simulink model "V1"  (R2025a)
settings: Solver=VariableStepAuto  StartTime=0.0  StopTime=200  FixedStep=0.005  RelTol=1e-3
libraries: cstblocks x11, vrlib x10, slpidlib x9, simulink_extras x8, dspinverses x3, robotcorelib x2, simulink x1
(part 1 of 3)
settings Model: Creator=HyeonMin  LastModifiedBy=user
settings SolverCC: AlgebraicLoopSolver=TrustRegion
settings DebuggingCC: UnderSpecifiedDimensionMsg=warning
settings RTWCC: GPUComputeCapability=3.5

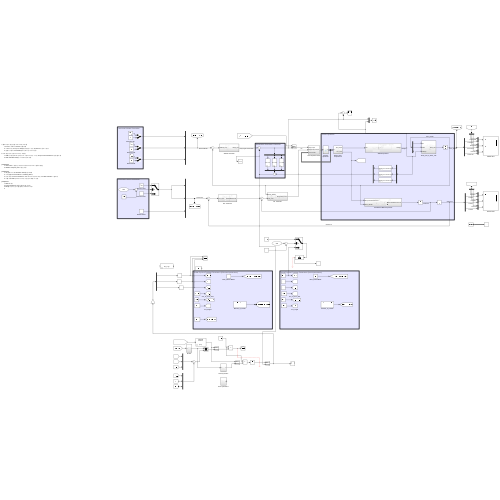
[thumbnail: Simulink's stored preview of the top-level diagram]
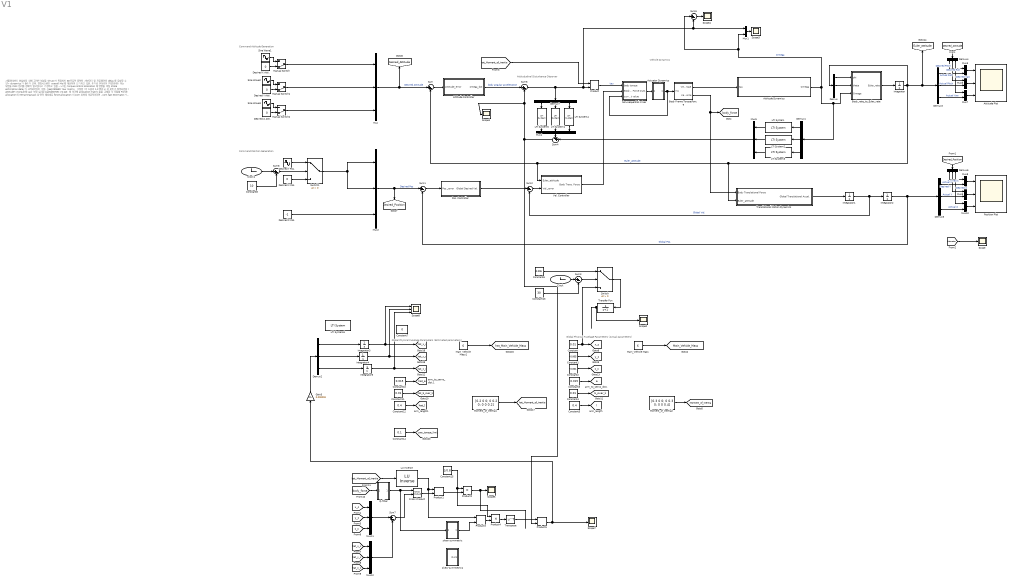
== system V1 ==
  note: Attitududinal Disturbance Observer
  note: Command Attitude Generation
  note: Command Position Generation
  note: 시뮬레이션의 현실성을 위해 고려한 부분들
      | thrust가 목표치의 80프로만 출력됨
      | 서보모터 및 프로펠러에 delay를 유발할 수 있는 dynamics가 들어가 있음.
      | 결합시스템의 overall MoI를 계산하여 인가하고 있음.
      |
      | 추가로 현실성이 반영되어야 하는 부분들
      | CoM 텐서를 정확히 알고있다고 가정하고 있음. ->이는 torque control allocation에 영향을 미침
      | state estimation delay가 고려되어있지 않음.
      |
      | [Jae]230630:
      | Yaw matrix 수정함 (각 드론의 1,2행의 xi 값 부호가 잘못되었음)
      | attitude->torque에 yaw 보정 실시함
      |
      | [Jae]230705:
      | V2 ppt에 의거해 allocation matrix들을 교체함
      | 각 모듈별 Force allocation이 remaining task임
      | 만약 예상대로 force allocation이 com 위치에 의존적이라면, com fast estimator가 필요함
      | 이를 위해 DOB 신호에 의거하는 것을 생각해볼 수 있음.
      |
      | [Jae]230731:
      | DOB 추가함.
      | torque allocation을 J를 곱함으로써 추가함.
      | MoI를 계산하는 공식을 물리량 파트에 추가함.
  note: Global Physical Fuselage Parameters (Actual parameters)
  note: Vehicle Dynamics
  note: Global Physical Fuselage Parameters (Estimated parameters)
  " LU Inverse" : dspinverses/ LU Inverse
  Actuator Dynamics : Subsystem
  Attitude Controller : Subsystem
  Attitude Dynamics : Subsystem
  Attitude Plot : Scope  NumInputPorts=3
      settings: Title=Fuselage Euler Attitude  ActiveDisplayYMinimum=-0.24923  ActiveDisplayYMaximum=0.11713  YLabel=Roll
  Body Frame Torque/Force : Subsystem
  Body_rate_to_Euler_rate : Subsystem
  Clock : Clock
  Clock1 : Clock
  Constant : Constant  Value=0.01
  Constant1 : Constant  Value=-0.005
  Constant10 : Constant  Value=0.015
  Constant11 : Constant  Value=0.01
  Constant12 : Constant  Value=0.4
  Constant13 : Constant  Value=30
  Constant14 : Constant  Value=0.1
  Constant15 : Constant  Value=1/0.8
  Constant2 : Constant  Value=-0.001
  Constant3 : Constant  Value=0.015
  Constant4 : Constant  Value=0.01
  Constant5 : Constant  Value=0.4
  Constant6 : Constant  Value=0.005
  Constant7 : Constant  Value=0
  Constant8 : Constant  Value=10
  Cross Product : vrlib/Utilities/Cross Product
  Demux{,1..7} (8 alike) : Demux  Outputs=3
  Desired X Atti. : Constant  Value=0
  Desired X Pos. : Constant  Value=0
  Desired Y Atti. : Constant  Value=0
  Desired Y Pos. : Sin  Amplitude=10  Frequency=0.5  SampleTime=0
  Desired Z Atti. : Constant  Value=0
  Desired Z Pos. : Constant  Value=-1
  Gain3 : Gain  Gain=0.000003
  Integrator{,1..5} (6 alike) : Integrator
  LTI System : cstblocks/LTI System  sys=tf([1 0],[1/1 1.414/1 1])  IC=[]  PadeOrder=0
  LTI System1 : cstblocks/LTI System  sys=tf([1],[1/1 1.414/1 1])  IC=[]  PadeOrder=0
  LTI System2 : cstblocks/LTI System  sys=tf([1 0],[1/1 1.414/1 1])  IC=[]  PadeOrder=0
  LTI System3 : cstblocks/LTI System  sys=tf([1 0],[1/1 1.414/1 1])  IC=[]  PadeOrder=0
  LTI System4 : cstblocks/LTI System  sys=tf([1],[1/1 1.414/1 1])  IC=[]  PadeOrder=0
  LTI System5 : cstblocks/LTI System  sys=tf([1],[1/1 1.414/1 1])  IC=[]  PadeOrder=0
  LTI System6 : cstblocks/LTI System  sys=tf(1,[1 1])  IC=[]  PadeOrder=0
  Main_Vehicle Mass : Constant  Value=6
  Main_Vehicle Mass1 : Constant  Value=6
  Manual Switch : ManualSwitch  CurrentSetting=0
  Manual Switch1 : ManualSwitch  CurrentSetting=0
  Manual Switch2 : ManualSwitch  CurrentSetting=0
  Moment_of_Inertia1 : Constant  Value=[0.2 0 0; 0 0.2 0; 0 0 0.2]  VectorParams1D=off
  Moment_of_Inertia2 : Constant  Value=[0.3 0 0; 0 0.3 0; 0 0 0.4]  VectorParams1D=off
  Mux{,2,4..5,11..12} (6 alike) : Mux  Inputs=3
  Mux{1,3,6..10} (7 alike) : Mux  Inputs=2
  Non-sequential mixer : Subsystem
  Pos. Controller : Subsystem
  Position Plot : Scope  NumInputPorts=3
      settings: Title=Fuselage Global Position  ActiveDisplayYMinimum=-12.5  ActiveDisplayYMaximum=12.5  YLabel=X Pos.
  Product{,1,3,5} (4 alike) : Product  Multiplication=Matrix(*)
  Product2 : Product
  Product4 : Product
  Q-filter : Subsystem
  Scope{,1..5,7} (7 alike) : Scope
      Scope settings: ActiveDisplayYMinimum=-12.2499  ActiveDisplayYMaximum=102.16663  DataLoggingVariableName=ScopeData2
      Scope1 settings: ActiveDisplayYMinimum=-1.84038  ActiveDisplayYMaximum=0.46914
      Scope2 settings: ActiveDisplayYMinimum=-0.00062  ActiveDisplayYMaximum=0.00562  DataLoggingVariableName=ScopeData7
      Scope3 settings: ActiveDisplayYMinimum=-16.98597  ActiveDisplayYMaximum=13.16908  DataLoggingVariableName=ScopeData2
      Scope4 settings: ActiveDisplayYMinimum=-12.97439  ActiveDisplayYMaximum=18.15104  DataLoggingVariableName=ScopeData3
      Scope5 settings: ActiveDisplayYMinimum=-11.747663892139656  ActiveDisplayYMaximum=3.3030131405781913  DataLoggingVariableName=ScopeData4
      Scope7 settings: ActiveDisplayYMinimum=-1130.28192  ActiveDisplayYMaximum=1419.66244  DataLoggingVariableName=ScopeData6
  Scope8 : Scope  NumInputPorts=3
      settings: ActiveDisplayYMinimum=-0.00763  ActiveDisplayYMaximum=0.01321  DataLoggingVariableName=ScopeData7
  Sine Wave1 : Sin  Amplitude=0.2  Frequency=0.4  SampleTime=0
  Sine Wave2 : Sin  Amplitude=0.2  Frequency=0.4  SampleTime=0
  Sine Wave3 : Sin  Frequency=0.2  SampleTime=0
  Sum{,1..3,5..8} (8 alike) : Sum  Inputs=|+-
  Sum4 : Sum  Inputs=-+|
  Switch : Switch  Criteria=u2 > Threshold  SaturateOnIntegerOverflow=off  InputSameDT=off
  Switch1 : Switch  Criteria=u2 > Threshold  SaturateOnIntegerOverflow=off  InputSameDT=off
  Transfer Fcn : TransferFcn  Denominator=[1 1]
  Translational Motion Dynamics : Subsystem
  Transpose : Math  Operator=transpose
  Vel. Controller : Subsystem
  skew-symmetric : Subsystem
  skew-symmetric1 : Subsystem
  tag scope: Desired_Attitude=global, Desired_Position=global, Euler_attitude=global, Main_Vehicle_Mass=global, Moment_of_Inertia=global, a=global, b_over_k=global, body_force=global, hat_Main_Vehicle_Mass=global, hat_Moment_of_Inertia=global, hat_a=global, hat_b_over_k=global, hat_l=global, hat_x_c=global, hat_y_c=global, hat_z_c=global, l=global, x_c=global, y_c=global, yaw_torque_limit=global, z_c=global
  wires:
  Mux/1 -> Sum/1, [Desired_Attitude]  "Desired Attitude"
  Sum/1 -> Attitude Controller/1(Attitude_error)
  Mux2/1 -> Sum1/1, [Desired_Position]  "Desired Pos"
  Desired Z Pos./1 -> Mux2/3
  Sum1/1 -> Pos. Controller/1(Pos._error)
  Pos. Controller/1(Global Desired Vel.) -> Sum2/1
  Sum2/1 -> Vel. Controller/2(Vel._error)
  Constant/1 -> [x_c], Switch/3
  Constant1/1 -> [y_c]
  Constant2/1 -> [z_c]
  Constant3/1 -> [a]
  Constant4/1 -> [b_over_k]
  Constant5/1 -> [l]
  Main_Vehicle Mass/1 -> [Main_Vehicle_Mass]
  Non-sequential mixer/1(Out1) -> Actuator Dynamics/1(In1)
  Integrator/1 -> Translational Motion Dynamics/2(Euler_attitude), Sum/2, Vel. Controller/1(Euler_attitude), [Euler_attitude], Demux3/1, Demux/1  "Euler_attitude"
  Demux/2 -> Body_rate_to_Euler_rate/2(theta)
  Demux/1 -> Body_rate_to_Euler_rate/1(phi)
  Demux4/1 -> Mux3/1  "Desired Roll"
  Demux4/2 -> Mux6/1  "Desired Pitch"
  [Desired_Attitude] -> Demux4/1
  Demux3/3 -> Mux7/2  "Actual Yaw"
  Demux3/1 -> Mux3/2  "Actual Roll"
  Demux3/2 -> Mux6/2  "Actual Pitch"
  Demux4/3 -> Mux7/1  "Desired Yaw"
  Mux3/1 -> Attitude Plot/1
  Mux6/1 -> Attitude Plot/2
  Mux7/1 -> Attitude Plot/3
  Body Frame Torque/Force/2(Vec_force) -> [body_force], Translational Motion Dynamics/1(Body Translational Force)
  Demux6/1 -> Mux8/1  "Desired X"
  Demux5/3 -> Mux10/2  "Actual Z"
  [Desired_Position] -> Demux6/1
  Mux9/1 -> Position Plot/2
  Demux6/3 -> Mux10/1  "Desired Z"
  Demux6/2 -> Mux9/1  "Desired Y"
  Demux5/1 -> Mux8/2  "Actual X"
  [Actuator] -> Scope/1
  Demux5/2 -> Mux9/2  "Actual Y"
  Mux8/1 -> Position Plot/1
  Integrator2/1 -> Sum1/2, Demux5/1  "Global Pos."
  Mux10/1 -> Position Plot/3
  Translational Motion Dynamics/1(Global Translational Accel.) -> Integrator1/1
  Integrator1/1 -> Sum2/2, Integrator2/1  "Global Vel."
  Sine Wave1/1 -> Manual Switch/1
  Manual Switch/1 -> Mux/1
  Sine Wave3/1 -> Manual Switch2/1
  Manual Switch2/1 -> Mux/3
  Desired X Atti./1 -> Manual Switch/2
  Sine Wave2/1 -> Manual Switch1/1
  Desired Y Atti./1 -> Manual Switch1/2
  Desired Z Atti./1 -> Manual Switch2/2
  Manual Switch1/1 -> Mux/2
  Attitude Dynamics/1(Omega) -> Sum5/1, Mux1/2, Demux1/1, Body_rate_to_Euler_rate/3(Omega)  "Omega"
  Actuator Dynamics/1(Out1) -> Non-sequential mixer/3(current value), Body Frame Torque/Force/1(In1)
  Main_Vehicle Mass1/1 -> [hat_Main_Vehicle_Mass]
  Constant12/1 -> [hat_l]
  Demux2/3 -> Integrator5/1
  Demux2/1 -> Integrator3/1
  Demux2/2 -> Integrator4/1
  Constant11/1 -> [hat_b_over_k]
  Constant10/1 -> [hat_a]
  Body Frame Torque/Force/1(Vec_torque) -> Attitude Dynamics/1(tau)
  Sum6/1 -> Sum5/2, Mux1/1, Product/2, Demux7/1
  Vel. Controller/1(Body Trans. Force) -> Non-sequential mixer/2(Body Trans. Force)
  Constant14/1 -> [yaw_torque_limit]
  [hat_Moment_of_Inertia] -> Product/1
  Product/1 -> Non-sequential mixer/1(body torque)  "tau"
  Attitude Controller/1(omega_dot) -> Sum6/1  "body angular acceleration"
  Moment_of_Inertia1/1 -> [hat_Moment_of_Inertia]
  Moment_of_Inertia2/1 -> [Moment_of_Inertia]
  Constant6/1 -> Switch/1
  Switch/1 -> Transfer Fcn/1
  Clock/1 -> Sum3/1
  Constant13/1 -> Sum3/2
  Sum3/1 -> Switch/2
  Transfer Fcn/1 -> Scope2/1
  Switch1/1 -> Mux2/2, Mux2/1
  Mux5/1 -> Sum4/2
  Mux4/1 -> Sum4/1
  Demux1/2 -> LTI System2/1
  Demux1/1 -> LTI System/1
  Demux1/3 -> LTI System3/1
  LTI System2/1 -> Mux5/2
  LTI System/1 -> Mux5/1
  LTI System3/1 -> Mux5/3
  Demux7/1 -> LTI System5/1
  Demux7/2 -> LTI System1/1
  Demux7/3 -> LTI System4/1
  LTI System1/1 -> Mux4/2
  Body_rate_to_Euler_rate/1(Euler_rate) -> Integrator/1
  Mux1/1 -> Scope3/1
  LTI System5/1 -> Mux4/1
  LTI System4/1 -> Mux4/3
  Sum5/1 -> Scope4/1
  [x_c] -> Mux11/1
  [y_c] -> Mux11/2
  [z_c] -> Mux11/3
  [hat_z_c] -> Mux12/3
  [hat_y_c] -> Mux12/2
  [hat_x_c] -> Mux12/1
  Mux12/1 -> Sum7/2
  Mux11/1 -> Sum7/1
  Sum7/1 -> Cross Product/2
  [body_force] -> Q-filter/1(In1)
  [hat_Moment_of_Inertia] -> " LU Inverse"/1
  " LU Inverse"/1 -> Product3/1, Product1/1
  Product1/1 -> Product2/2
  Constant15/1 -> Product4/1, Product2/1
  Cross Product/1 -> Product1/2
  Product2/1 -> Scope5/1
  skew-symmetric/1(Out1) -> Product3/2
  Product3/1 -> Product4/2
  Product4/1 -> Transpose/1
  Transpose/1 -> Product5/1
  Product5/1 -> Gain3/1, Scope7/1
  Sum4/1 -> Product5/2, Scope1/1, Sum6/2
  Q-filter/1(Out1) -> skew-symmetric/1(In1), Cross Product/1
  Integrator3/1 -> [hat_x_c], Scope8/1
  Integrator4/1 -> [hat_y_c], Scope8/2
  Integrator5/1 -> [hat_z_c], Scope8/3
  Gain3/1 -> Demux2/1
  Clock1/1 -> Sum8/1
  Sum8/1 -> Switch1/2
  Desired X Pos./1 -> Switch1/3
  Constant8/1 -> Sum8/2
  Desired Y Pos./1 -> Switch1/1

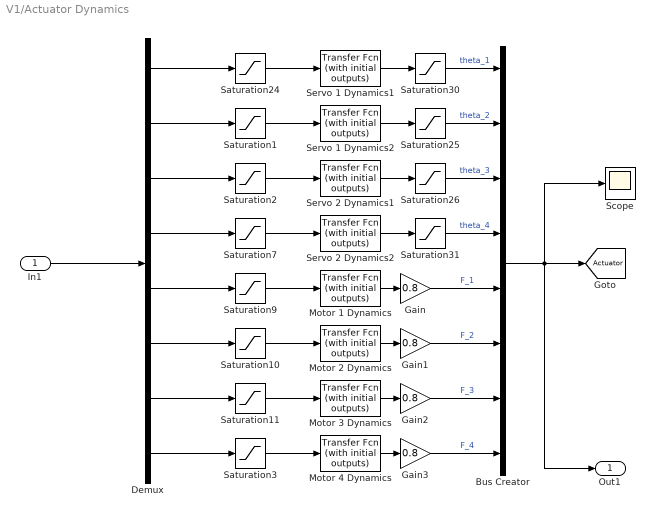
== system V1/Actuator Dynamics ==
  In1 : Inport
  Bus Creator : BusCreator  Inputs=8
  Demux : Demux  Outputs=8
  Gain{,1..3} (4 alike) : Gain  Gain=0.8
  Motor 1 Dynamics : simulink_extras/Additional Linear/Transfer Fcn (with initial outputs)  N=[1]  D="[1/100  1]"  Y0=0  U0=0
  Motor 2 Dynamics : simulink_extras/Additional Linear/Transfer Fcn (with initial outputs)  N=[1]  D="[1/100  1]"  Y0=0  U0=0
  Motor 3 Dynamics : simulink_extras/Additional Linear/Transfer Fcn (with initial outputs)  N=[1]  D="[1/100  1]"  Y0=0  U0=0
  Motor 4 Dynamics : simulink_extras/Additional Linear/Transfer Fcn (with initial outputs)  N=[1]  D="[1/100  1]"  Y0=0  U0=0
  Saturation{1..2,7,24..26,30..31} (8 alike) : Saturate  UpperLimit=1  LowerLimit=-1
  Saturation{3,9..11} (4 alike) : Saturate  UpperLimit=200  LowerLimit=0
  Scope : Scope
      settings: ActiveDisplayYMinimum=-0.77379  ActiveDisplayYMaximum=0.4348  DataLoggingVariableName=ScopeData8
  Servo 1 Dynamics1 : simulink_extras/Additional Linear/Transfer Fcn (with initial outputs)  N=[1]  D="[1/30  1]"  Y0=0  U0=0
  Servo 1 Dynamics2 : simulink_extras/Additional Linear/Transfer Fcn (with initial outputs)  N=[1]  D="[1/30  1]"  Y0=0  U0=0
  Servo 2 Dynamics1 : simulink_extras/Additional Linear/Transfer Fcn (with initial outputs)  N=[1]  D="[1/30  1]"  Y0=0  U0=0
  Servo 2 Dynamics2 : simulink_extras/Additional Linear/Transfer Fcn (with initial outputs)  N=[1]  D="[1/30  1]"  Y0=0  U0=0
  Out1 : Outport
  tag scope: Actuator=global
  wires:
  Demux/6 -> Saturation10/1
  Demux/7 -> Saturation11/1
  Demux/8 -> Saturation3/1
  Bus Creator/1 -> Out1/1, [Actuator], Scope/1
  Gain/1 -> Bus Creator/5  "F_1"
  Gain1/1 -> Bus Creator/6  "F_2"
  Gain2/1 -> Bus Creator/7  "F_3"
  Gain3/1 -> Bus Creator/8  "F_4"
  Servo 2 Dynamics1/1 -> Saturation26/1
  Servo 2 Dynamics2/1 -> Saturation31/1
  Saturation2/1 -> Servo 2 Dynamics1/1
  Saturation7/1 -> Servo 2 Dynamics2/1
  Saturation9/1 -> Motor 1 Dynamics/1
  Saturation10/1 -> Motor 2 Dynamics/1
  Saturation11/1 -> Motor 3 Dynamics/1
  Saturation3/1 -> Motor 4 Dynamics/1
  Saturation1/1 -> Servo 1 Dynamics2/1
  Servo 1 Dynamics2/1 -> Saturation25/1
  Saturation24/1 -> Servo 1 Dynamics1/1
  Servo 1 Dynamics1/1 -> Saturation30/1
  Demux/5 -> Saturation9/1
  Demux/2 -> Saturation1/1
  Demux/1 -> Saturation24/1
  Demux/3 -> Saturation2/1
  Demux/4 -> Saturation7/1
  Saturation30/1 -> Bus Creator/1  "theta_1"
  Saturation25/1 -> Bus Creator/2  "theta_2"
  Saturation26/1 -> Bus Creator/3  "theta_3"
  Saturation31/1 -> Bus Creator/4  "theta_4"
  Motor 1 Dynamics/1 -> Gain/1
  Motor 2 Dynamics/1 -> Gain1/1
  Motor 3 Dynamics/1 -> Gain2/1
  Motor 4 Dynamics/1 -> Gain3/1
  In1/1 -> Demux/1

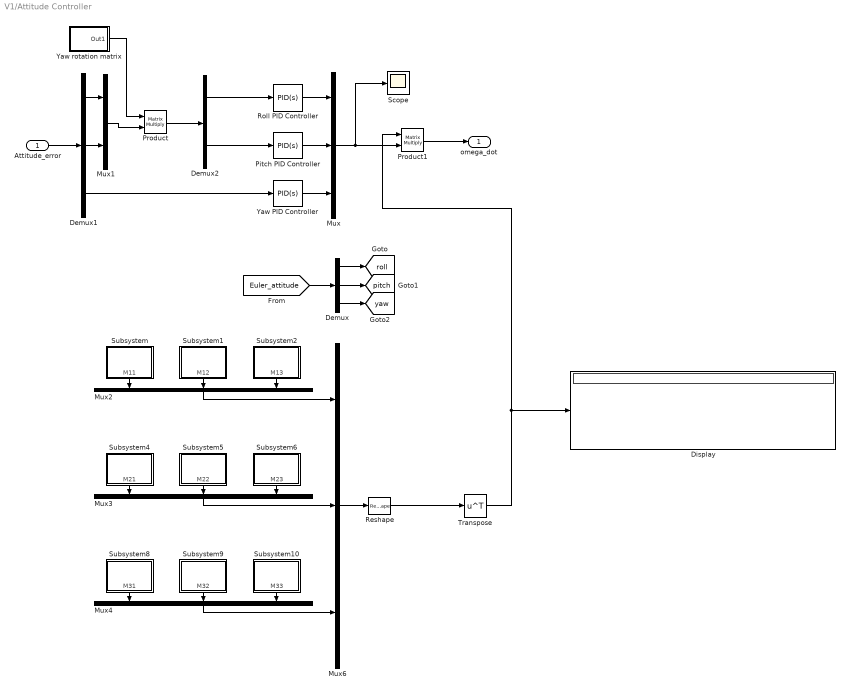
== system V1/Attitude Controller ==
  Attitude_error : Inport
  Demux : Demux  Outputs=3
  Demux1 : Demux  Outputs=3
  Demux2 : Demux  Outputs=2
  Display : Display
  Mux{,2..4,6} (5 alike) : Mux  Inputs=3
  Mux1 : Mux  Inputs=2
  Pitch PID Controller : slpidlib/PID Controller  Controller=PID  Form=Parallel  TimeDomain=Continuous-time  UseExternalTs=off  SampleTime=-1  IntegratorMethod=Forward Euler  FilterMethod=Forward Euler  ControllerParametersSource=internal  P=10  I=0  UseKiTs=off  D=3  UseExternalDerivativeSource=off  N=100  UseFilter=on  TunerSelectOption=Transfer Function Based (PID Tuner App)  InitialConditionSource=internal  InitialConditionForIntegrator=0  InitialConditionForFilter=0  DifferentiatorICPrevScaledInput=0  ExternalReset=none  TrackingMode=off  Kt=1  LimitOutput=off  SatLimitsSource=internal  UpperSaturationLimit=inf  LowerSaturationLimit=-inf  LinearizeAsGain=on  AntiWindupMode=none  Kb=1  LimitIntegrator=off  UpperIntegratorSaturationLimit=inf  LowerIntegratorSaturationLimit=-inf  POutMin=[]  POutMax=[]  IOutMin=[]  IOutMax=10  DOutMin=[]  DOutMax=[]  NOutMin=[]  NOutMax=[]  SumOutMin=[]  SumOutMax=[]  SaturationOutMin=[]  SaturationOutMax=[]  PParamMin=[]  PParamMax=[]  IParamMin=[]  IParamMax=[]  DParamMin=[]  DParamMax=[]  NParamMin=[]  NParamMax=[]  KbParamMin=[]  KbParamMax=[]  KtParamMin=[]  KtParamMax=[]  KbOutMin=[]  KbOutMax=[]  KtOutMin=[]  KtOutMax=[]  IntegratorOutMin=[]  IntegratorOutMax=[]  FilterOutMin=[]  FilterOutMax=[]  SumI1OutMin=[]  SumI1OutMax=[]  SumI2OutMin=[]  SumI2OutMax=[]  SumI3OutMin=[]  SumI3OutMax=[]  SumI4OutMin=[]  SumI4OutMax=[]  SumDOutMin=[]  SumDOutMax=[]  DifferentiatorOutMin=[]  DifferentiatorOutMax=[]  FilterDiffOutCoefMin=[]  FilterDiffOutCoefMax=[]  ReciprocalOutMin=[]  ReciprocalOutMax=[]  SumDenOutMin=[]  SumDenOutMax=[]  SumNumOutMin=[]  SumNumOutMax=[]  DivideOutMin=[]  DivideOutMax=[]  UdiffTsProdOutMin=[]  UdiffTsProdOutMax=[]  NTsProdOutMin=[]  NTsProdOutMax=[]  UintegralTsProdOutMin=[]  UintegralTsProdOutMax=[]  UngainTsProdOutMin=[]  UngainTsProdOutMax=[]  ClampingZeroOutDataTypeStr=Inherit: Inherit via back propagation  ClampingZeroOutMin=[]  ClampingZeroOutMax=[]  FilterDenConstantOutDataTypeStr=Inherit: Inherit via back propagation  FilterDenConstantOutMin=[]  FilterDenConstantOutMax=[]  PCopyOutDataTypeStr=Inherit: Inherit via back propagation  PCopyOutMin=[]  PCopyOutMax=[]  NCopyOutDataTypeStr=Inherit: Inherit via back propagation  NCopyOutMin=[]  NCopyOutMax=[]  IntegratorContinuousStateAttributes=''  IntegratorStateMustResolveToSignalObject=off  IntegratorRTWStateStorageClass=Auto  FilterContinuousStateAttributes=''  FilterStateMustResolveToSignalObject=off  FilterRTWStateStorageClass=Auto  ParallelPVariant=InternalParameters  IdealPVariant=Disabled  IVariant=InternalParameters  DVariant=InternalParameters  IntegratorVariant=Continuous  SatVariant=Disabled  AWVariant=Passthrough  PCopyVariant=Disabled  TRVariant=Disabled  FdbkBlocksVariant=Forward  IdealPFdbkVariant=Disabled  SatFdbkVariant=Disabled  DerivativeFilterVariant=ContFilter  NVariant=InternalParameters  NCopyVariant=Disabled  FilterICVariant=InternalICsFilter  IntegratorICVariant=InternalICs  ExternalResetVariant=Disabled  TRSumVariant=Passthrough  SumFdbkVariant=Disabled  SumVariant=Sum_PID  TsampFilterVariant=InternalTs  TsampNgainVariant=Passthrough  TsampIntegralVariant=Disabled_SignalSpec  ExternalSaturationOutDataTypeStr=Inherit: Same as second input  DerivativeSourceVariant=ErrorSignal  PreIntVariant=InternalPreInt
  Product : Product  Multiplication=Matrix(*)
  Product1 : Product  Multiplication=Matrix(*)
  Reshape : Reshape  OutputDimensionality=Customize  OutputDimensions=[3,3]
  Roll PID Controller : slpidlib/PID Controller  Controller=PID  Form=Parallel  TimeDomain=Continuous-time  UseExternalTs=off  SampleTime=-1  IntegratorMethod=Forward Euler  FilterMethod=Forward Euler  ControllerParametersSource=internal  P=10  I=0  UseKiTs=off  D=3  UseExternalDerivativeSource=off  N=100  UseFilter=on  TunerSelectOption=Transfer Function Based (PID Tuner App)  InitialConditionSource=internal  InitialConditionForIntegrator=0  InitialConditionForFilter=0  DifferentiatorICPrevScaledInput=0  ExternalReset=none  TrackingMode=off  Kt=1  LimitOutput=off  SatLimitsSource=internal  UpperSaturationLimit=inf  LowerSaturationLimit=-inf  LinearizeAsGain=on  AntiWindupMode=none  Kb=1  LimitIntegrator=off  UpperIntegratorSaturationLimit=inf  LowerIntegratorSaturationLimit=-inf  POutMin=[]  POutMax=[]  IOutMin=[]  IOutMax=[]  DOutMin=[]  DOutMax=[]  NOutMin=[]  NOutMax=[]  SumOutMin=[]  SumOutMax=[]  SaturationOutMin=[]  SaturationOutMax=[]  PParamMin=[]  PParamMax=[]  IParamMin=[]  IParamMax=[]  DParamMin=[]  DParamMax=[]  NParamMin=[]  NParamMax=[]  KbParamMin=[]  KbParamMax=[]  KtParamMin=[]  KtParamMax=[]  KbOutMin=[]  KbOutMax=[]  KtOutMin=[]  KtOutMax=[]  IntegratorOutMin=[]  IntegratorOutMax=[]  FilterOutMin=[]  FilterOutMax=[]  SumI1OutMin=[]  SumI1OutMax=[]  SumI2OutMin=[]  SumI2OutMax=[]  SumI3OutMin=[]  SumI3OutMax=[]  SumI4OutMin=[]  SumI4OutMax=[]  SumDOutMin=[]  SumDOutMax=[]  DifferentiatorOutMin=[]  DifferentiatorOutMax=[]  FilterDiffOutCoefMin=[]  FilterDiffOutCoefMax=[]  ReciprocalOutMin=[]  ReciprocalOutMax=[]  SumDenOutMin=[]  SumDenOutMax=[]  SumNumOutMin=[]  SumNumOutMax=[]  DivideOutMin=[]  DivideOutMax=[]  UdiffTsProdOutMin=[]  UdiffTsProdOutMax=[]  NTsProdOutMin=[]  NTsProdOutMax=[]  UintegralTsProdOutMin=[]  UintegralTsProdOutMax=[]  UngainTsProdOutMin=[]  UngainTsProdOutMax=[]  ClampingZeroOutDataTypeStr=Inherit: Inherit via back propagation  ClampingZeroOutMin=[]  ClampingZeroOutMax=[]  FilterDenConstantOutDataTypeStr=Inherit: Inherit via back propagation  FilterDenConstantOutMin=[]  FilterDenConstantOutMax=[]  PCopyOutDataTypeStr=Inherit: Inherit via back propagation  PCopyOutMin=[]  PCopyOutMax=[]  NCopyOutDataTypeStr=Inherit: Inherit via back propagation  NCopyOutMin=[]  NCopyOutMax=[]  IntegratorContinuousStateAttributes=''  IntegratorStateMustResolveToSignalObject=off  IntegratorRTWStateStorageClass=Auto  FilterContinuousStateAttributes=''  FilterStateMustResolveToSignalObject=off  FilterRTWStateStorageClass=Auto  ParallelPVariant=InternalParameters  IdealPVariant=Disabled  IVariant=InternalParameters  DVariant=InternalParameters  IntegratorVariant=Continuous  SatVariant=Disabled  AWVariant=Passthrough  PCopyVariant=Disabled  TRVariant=Disabled  FdbkBlocksVariant=Forward  IdealPFdbkVariant=Disabled  SatFdbkVariant=Disabled  DerivativeFilterVariant=ContFilter  NVariant=InternalParameters  NCopyVariant=Disabled  FilterICVariant=InternalICsFilter  IntegratorICVariant=InternalICs  ExternalResetVariant=Disabled  TRSumVariant=Passthrough  SumFdbkVariant=Disabled  SumVariant=Sum_PID  TsampFilterVariant=InternalTs  TsampNgainVariant=Passthrough  TsampIntegralVariant=Disabled_SignalSpec  ExternalSaturationOutDataTypeStr=Inherit: Same as second input  DerivativeSourceVariant=ErrorSignal  PreIntVariant=InternalPreInt
  Scope : Scope
      settings: ActiveDisplayYMinimum=-5.5328  ActiveDisplayYMaximum=0.61476  DataLoggingVariableName=ScopeData2
  Subsystem : Subsystem
  Subsystem1 : Subsystem
  Subsystem10 : Subsystem
  Subsystem2 : Subsystem
  Subsystem4 : Subsystem
  Subsystem5 : Subsystem
  Subsystem6 : Subsystem
  Subsystem8 : Subsystem
  Subsystem9 : Subsystem
  Transpose : Math  Operator=transpose
  Yaw PID Controller : slpidlib/PID Controller  Controller=PID  Form=Parallel  TimeDomain=Continuous-time  UseExternalTs=off  SampleTime=-1  IntegratorMethod=Forward Euler  FilterMethod=Forward Euler  ControllerParametersSource=internal  P=10  I=0  UseKiTs=off  D=3  UseExternalDerivativeSource=off  N=100  UseFilter=on  TunerSelectOption=Transfer Function Based (PID Tuner App)  InitialConditionSource=internal  InitialConditionForIntegrator=0  InitialConditionForFilter=0  DifferentiatorICPrevScaledInput=0  ExternalReset=none  TrackingMode=off  Kt=1  LimitOutput=off  SatLimitsSource=internal  UpperSaturationLimit=1  LowerSaturationLimit=-1  LinearizeAsGain=on  AntiWindupMode=none  Kb=1  LimitIntegrator=off  UpperIntegratorSaturationLimit=inf  LowerIntegratorSaturationLimit=-inf  POutMin=[]  POutMax=[]  IOutMin=[]  IOutMax=10  DOutMin=[]  DOutMax=[]  NOutMin=[]  NOutMax=[]  SumOutMin=[]  SumOutMax=[]  SaturationOutMin=[]  SaturationOutMax=[]  PParamMin=[]  PParamMax=[]  IParamMin=[]  IParamMax=[]  DParamMin=[]  DParamMax=[]  NParamMin=[]  NParamMax=[]  KbParamMin=[]  KbParamMax=[]  KtParamMin=[]  KtParamMax=[]  KbOutMin=[]  KbOutMax=[]  KtOutMin=[]  KtOutMax=[]  IntegratorOutMin=[]  IntegratorOutMax=[]  FilterOutMin=[]  FilterOutMax=[]  SumI1OutMin=[]  SumI1OutMax=[]  SumI2OutMin=[]  SumI2OutMax=[]  SumI3OutMin=[]  SumI3OutMax=[]  SumI4OutMin=[]  SumI4OutMax=[]  SumDOutMin=[]  SumDOutMax=[]  DifferentiatorOutMin=[]  DifferentiatorOutMax=[]  FilterDiffOutCoefMin=[]  FilterDiffOutCoefMax=[]  ReciprocalOutMin=[]  ReciprocalOutMax=[]  SumDenOutMin=[]  SumDenOutMax=[]  SumNumOutMin=[]  SumNumOutMax=[]  DivideOutMin=[]  DivideOutMax=[]  UdiffTsProdOutMin=[]  UdiffTsProdOutMax=[]  NTsProdOutMin=[]  NTsProdOutMax=[]  UintegralTsProdOutMin=[]  UintegralTsProdOutMax=[]  UngainTsProdOutMin=[]  UngainTsProdOutMax=[]  ClampingZeroOutDataTypeStr=Inherit: Inherit via back propagation  ClampingZeroOutMin=[]  ClampingZeroOutMax=[]  FilterDenConstantOutDataTypeStr=Inherit: Inherit via back propagation  FilterDenConstantOutMin=[]  FilterDenConstantOutMax=[]  PCopyOutDataTypeStr=Inherit: Inherit via back propagation  PCopyOutMin=[]  PCopyOutMax=[]  NCopyOutDataTypeStr=Inherit: Inherit via back propagation  NCopyOutMin=[]  NCopyOutMax=[]  IntegratorContinuousStateAttributes=''  IntegratorStateMustResolveToSignalObject=off  IntegratorRTWStateStorageClass=Auto  FilterContinuousStateAttributes=''  FilterStateMustResolveToSignalObject=off  FilterRTWStateStorageClass=Auto  ParallelPVariant=InternalParameters  IdealPVariant=Disabled  IVariant=InternalParameters  DVariant=InternalParameters  IntegratorVariant=Continuous  SatVariant=Disabled  AWVariant=Passthrough  PCopyVariant=Disabled  TRVariant=Disabled  FdbkBlocksVariant=Forward  IdealPFdbkVariant=Disabled  SatFdbkVariant=Disabled  DerivativeFilterVariant=ContFilter  NVariant=InternalParameters  NCopyVariant=Disabled  FilterICVariant=InternalICsFilter  IntegratorICVariant=InternalICs  ExternalResetVariant=Disabled  TRSumVariant=Passthrough  SumFdbkVariant=Disabled  SumVariant=Sum_PID  TsampFilterVariant=InternalTs  TsampNgainVariant=Passthrough  TsampIntegralVariant=Disabled_SignalSpec  ExternalSaturationOutDataTypeStr=Inherit: Same as second input  DerivativeSourceVariant=ErrorSignal  PreIntVariant=InternalPreInt
  Yaw rotation matrix : Subsystem
  omega_dot : Outport
  tag scope: pitch=global, roll=global, yaw=global
  wires:
  Demux1/1 -> Mux1/1
  Demux1/3 -> Yaw PID Controller/1
  Demux1/2 -> Mux1/2
  Pitch PID Controller/1 -> Mux/2
  Mux/1 -> Product1/2, Scope/1
  Attitude_error/1 -> Demux1/1
  Roll PID Controller/1 -> Mux/1
  Yaw rotation matrix/1(Out1) -> Product/1
  Mux1/1 -> Product/2
  Product/1 -> Demux2/1
  Demux2/1 -> Roll PID Controller/1
  Demux2/2 -> Pitch PID Controller/1
  Yaw PID Controller/1 -> Mux/3
  Reshape/1 -> Transpose/1
  Mux3/1 -> Mux6/2
  Transpose/1 -> Product1/1, Display/1
  Subsystem9/1(M32) -> Mux4/2
  Subsystem10/1(M33) -> Mux4/3
  Mux4/1 -> Mux6/3
  Subsystem/1(M11) -> Mux2/1
  Subsystem8/1(M31) -> Mux4/1
  Subsystem2/1(M13) -> Mux2/3
  Subsystem4/1(M21) -> Mux3/1
  Mux2/1 -> Mux6/1
  Mux6/1 -> Reshape/1
  Subsystem5/1(M22) -> Mux3/2
  Subsystem1/1(M12) -> Mux2/2
  Subsystem6/1(M23) -> Mux3/3
  [Euler_attitude] -> Demux/1
  Demux/1 -> [roll]
  Demux/2 -> [pitch]
  Demux/3 -> [yaw]
  Product1/1 -> omega_dot/1

== system V1/Attitude Dynamics ==
  note: J Omega_dot=tau-Omega X J Omega
      | Omega_dot=J^{-1} (tau-Omega X J Omega)
  tau : Inport
  Cross Product : vrlib/Utilities/Cross Product
  Divide : Product  Inputs=/*  Multiplication=Matrix(*)
  Integrator : Integrator
  Product : Product  Multiplication=Matrix(*)
  Sum : Sum  Inputs=|+-
  Omega : Outport
  wires:
  Cross Product/1 -> Sum/2
  tau/1 -> Sum/1
  Sum/1 -> Divide/2
  Integrator/1 -> Product/2, Cross Product/1, Omega/1
  Product/1 -> Cross Product/2
  [Moment_of_Inertia] -> Divide/1, Product/1
  Divide/1 -> Integrator/1  "Omega_dot"

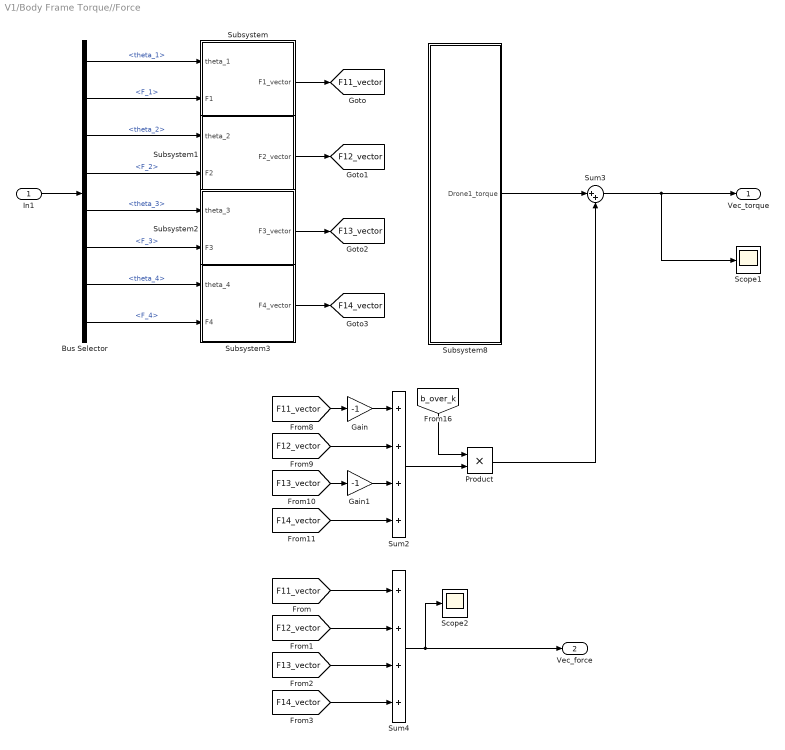
== system V1/Body Frame Torque//Force ==
  In1 : Inport
  Bus Selector : BusSelector  OutputSignals=theta_1,F_1,theta_2,F_2,theta_3,F_3,theta_4,F_4
  Gain : Gain  Gain=-1
  Gain1 : Gain  Gain=-1
  Product : Product
  Scope1 : Scope
      settings: ActiveDisplayYMinimum=-4.71618  ActiveDisplayYMaximum=3.68639  DataLoggingVariableName=ScopeData6
  Scope2 : Scope
      settings: ActiveDisplayYMinimum=-521.49261  ActiveDisplayYMaximum=88.4469  DataLoggingVariableName=ScopeData7
  Subsystem : Subsystem
  Subsystem1 : Subsystem
  Subsystem2 : Subsystem
  Subsystem3 : Subsystem
  Subsystem8 : Subsystem
  Sum2 : Sum  Inputs=++++
  Sum3 : Sum  Inputs=|++
  Sum4 : Sum  Inputs=++++
  Vec_torque : Outport
  Vec_force : Outport  Port=2
  tag scope: F11_vector=global, F12_vector=global, F13_vector=global, F14_vector=global
  wires:
  In1/1 -> Bus Selector/1
  Bus Selector/1 -> Subsystem/1(theta_1)  "<theta_1>"
  Bus Selector/2 -> Subsystem/2(F1)  "<F_1>"
  Bus Selector/3 -> Subsystem1/1(theta_2)  "<theta_2>"
  Bus Selector/4 -> Subsystem1/2(F2)  "<F_2>"
  Bus Selector/5 -> Subsystem2/1(theta_3)  "<theta_3>"
  Bus Selector/6 -> Subsystem2/2(F3)  "<F_3>"
  Bus Selector/7 -> Subsystem3/1(theta_4)  "<theta_4>"
  Bus Selector/8 -> Subsystem3/2(F4)  "<F_4>"
  Subsystem/1(F1_vector) -> [F11_vector]
  Subsystem1/1(F2_vector) -> [F12_vector]
  Subsystem2/1(F3_vector) -> [F13_vector]
  Subsystem3/1(F4_vector) -> [F14_vector]
  Sum3/1 -> Scope1/1, Vec_torque/1
  [F12_vector] -> Sum4/2
  [F11_vector] -> Sum4/1
  [F13_vector] -> Sum4/3
  [F14_vector] -> Sum4/4
  [F12_vector] -> Sum2/2
  [F13_vector] -> Gain1/1
  [F11_vector] -> Gain/1
  [F14_vector] -> Sum2/4
  Sum2/1 -> Product/2
  [b_over_k] -> Product/1
  Gain/1 -> Sum2/1
  Gain1/1 -> Sum2/3
  Subsystem8/1(Drone1_torque) -> Sum3/1
  Sum4/1 -> Vec_force/1, Scope2/1
  Product/1 -> Sum3/2

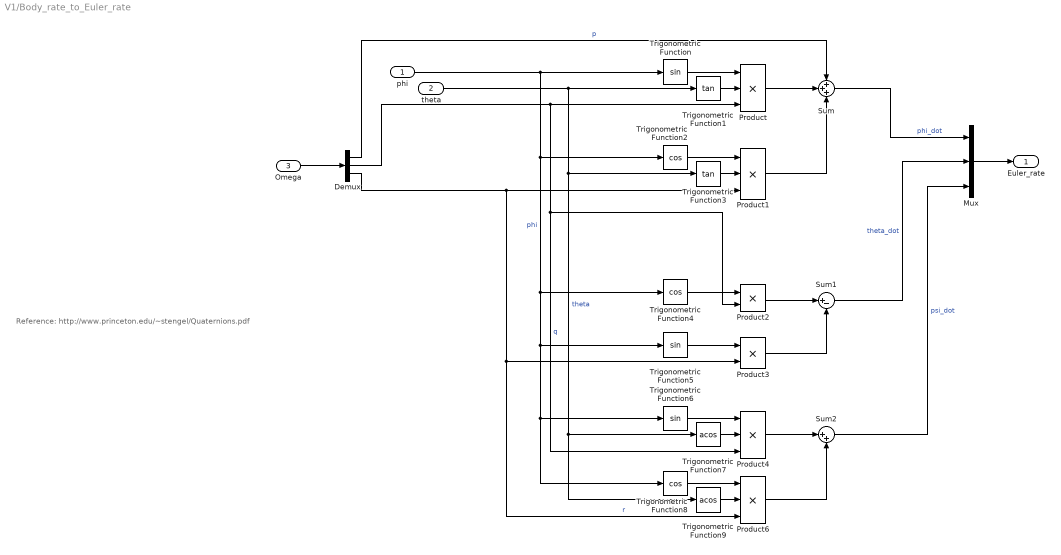
== system V1/Body_rate_to_Euler_rate ==
  note: Reference: http://www.princeton.edu/~stengel/Quaternions.pdf
  phi : Inport
  theta : Inport  Port=2
  Omega : Inport  Port=3
  Demux : Demux  Outputs=3
  Mux : Mux  Inputs=3
  Product{,1,4,6} (4 alike) : Product  Inputs=3
  Product2 : Product
  Product3 : Product
  Sum : Sum  Inputs=+++
  Sum1 : Sum  Inputs=|+-
  Sum2 : Sum  Inputs=|++
  Trigonometric Function : Trigonometry
  Trigonometric Function1 : Trigonometry  Operator=tan
  Trigonometric Function2 : Trigonometry  Operator=cos
  Trigonometric Function3 : Trigonometry  Operator=tan
  Trigonometric Function4 : Trigonometry  Operator=cos
  Trigonometric Function5 : Trigonometry
  Trigonometric Function6 : Trigonometry
  Trigonometric Function7 : Trigonometry  Operator=acos
  Trigonometric Function8 : Trigonometry  Operator=cos
  Trigonometric Function9 : Trigonometry  Operator=acos
  Euler_rate : Outport
  wires:
  phi/1 -> Trigonometric Function2/1, Trigonometric Function8/1, Trigonometric Function6/1, Trigonometric Function5/1, Trigonometric Function4/1, Trigonometric Function/1  "phi"
  Demux/3 -> Product6/3, Product3/2, Product1/3  "r"
  Trigonometric Function9/1 -> Product6/2
  theta/1 -> Trigonometric Function9/1, Trigonometric Function7/1, Trigonometric Function3/1, Trigonometric Function1/1  "theta"
  Trigonometric Function7/1 -> Product4/2
  Demux/2 -> Product4/3, Product2/2, Product/3  "q"
  Sum/1 -> Mux/1  "phi_dot"
  Product4/1 -> Sum2/1
  Trigonometric Function6/1 -> Product4/1
  Trigonometric Function5/1 -> Product3/1
  Product/1 -> Sum/2
  Product6/1 -> Sum2/2
  Product3/1 -> Sum1/2
  Product2/1 -> Sum1/1
  Trigonometric Function/1 -> Product/1
  Trigonometric Function4/1 -> Product2/1
  Trigonometric Function3/1 -> Product1/2
  Trigonometric Function1/1 -> Product/2
  Trigonometric Function8/1 -> Product6/1
  Trigonometric Function2/1 -> Product1/1
  Product1/1 -> Sum/3
  Sum1/1 -> Mux/2  "theta_dot"
  Sum2/1 -> Mux/3  "psi_dot"
  Demux/1 -> Sum/1  "p"
  Omega/1 -> Demux/1
  Mux/1 -> Euler_rate/1

== system V1/Non-sequential mixer ==
  body torque : Inport
  Body Trans. Force : Inport  Port=2
  current value : Inport  Port=3
  Bus Creator : BusCreator  Inputs=6
  Demux : Demux  Outputs=3
  Demux1 : Demux  Outputs=3
  Mux : Mux  Inputs=2
  Mux1 : Mux  Inputs=3
  Wrench allocation_Drone1 : Subsystem
  "[P1] Control allocation" : Subsystem
  Out1 : Outport
  tag scope: Sensor=global
  wires:
  current value/1 -> [Sensor]
  Demux/1 -> Bus Creator/1  "tau_x"
  Demux/2 -> Bus Creator/2  "tau_y"
  Demux/3 -> Bus Creator/3  "tau_z"
  body torque/1 -> Demux/1
  Demux1/1 -> Bus Creator/4  "F_x"
  Demux1/2 -> Bus Creator/5  "F_y"
  Demux1/3 -> Bus Creator/6  "F_z"
  Body Trans. Force/1 -> Demux1/1
  "[P1] Control allocation"/2("[P1] Servo angle command") -> Mux/1
  "[P1] Control allocation"/1("[P1] Motor thrust cmd") -> Mux/2
  Mux/1 -> Out1/1
  Bus Creator/1 -> Wrench allocation_Drone1/1(In1)  "Overall control wrench"
  Wrench allocation_Drone1/1(Out1) -> "[P1] Control allocation"/1(In1)
  [hat_x_c] -> Mux1/1
  [hat_y_c] -> Mux1/2
  [hat_z_c] -> Mux1/3
  Mux1/1 -> "[P1] Control allocation"/2("x_{c,p2}")

== system V1/Pos. Controller ==
  Pos._error : Inport
  Demux1 : Demux  Outputs=3
  Mux : Mux  Inputs=3
  Scope : Scope
      settings: ActiveDisplayYMinimum=-2.5  ActiveDisplayYMaximum=2.5  DataLoggingVariableName=ScopeData2
  X PID Controller : slpidlib/PID Controller  Controller=PID  Form=Parallel  TimeDomain=Continuous-time  UseExternalTs=off  SampleTime=-1  IntegratorMethod=Forward Euler  FilterMethod=Forward Euler  ControllerParametersSource=internal  P=2  I=0  UseKiTs=off  D=1  UseExternalDerivativeSource=off  N=100  UseFilter=on  TunerSelectOption=Transfer Function Based (PID Tuner App)  InitialConditionSource=internal  InitialConditionForIntegrator=0  InitialConditionForFilter=0  DifferentiatorICPrevScaledInput=0  ExternalReset=none  TrackingMode=off  Kt=1  LimitOutput=off  SatLimitsSource=internal  UpperSaturationLimit=2  LowerSaturationLimit=-2  LinearizeAsGain=on  AntiWindupMode=none  Kb=1  LimitIntegrator=off  UpperIntegratorSaturationLimit=inf  LowerIntegratorSaturationLimit=-inf  POutMin=[]  POutMax=[]  IOutMin=[]  IOutMax=10  DOutMin=[]  DOutMax=[]  NOutMin=[]  NOutMax=[]  SumOutMin=[]  SumOutMax=[]  SaturationOutMin=[]  SaturationOutMax=[]  PParamMin=[]  PParamMax=[]  IParamMin=[]  IParamMax=[]  DParamMin=[]  DParamMax=[]  NParamMin=[]  NParamMax=[]  KbParamMin=[]  KbParamMax=[]  KtParamMin=[]  KtParamMax=[]  KbOutMin=[]  KbOutMax=[]  KtOutMin=[]  KtOutMax=[]  IntegratorOutMin=[]  IntegratorOutMax=[]  FilterOutMin=[]  FilterOutMax=[]  SumI1OutMin=[]  SumI1OutMax=[]  SumI2OutMin=[]  SumI2OutMax=[]  SumI3OutMin=[]  SumI3OutMax=[]  SumI4OutMin=[]  SumI4OutMax=[]  SumDOutMin=[]  SumDOutMax=[]  DifferentiatorOutMin=[]  DifferentiatorOutMax=[]  FilterDiffOutCoefMin=[]  FilterDiffOutCoefMax=[]  ReciprocalOutMin=[]  ReciprocalOutMax=[]  SumDenOutMin=[]  SumDenOutMax=[]  SumNumOutMin=[]  SumNumOutMax=[]  DivideOutMin=[]  DivideOutMax=[]  UdiffTsProdOutMin=[]  UdiffTsProdOutMax=[]  NTsProdOutMin=[]  NTsProdOutMax=[]  UintegralTsProdOutMin=[]  UintegralTsProdOutMax=[]  UngainTsProdOutMin=[]  UngainTsProdOutMax=[]  ClampingZeroOutDataTypeStr=Inherit: Inherit via back propagation  ClampingZeroOutMin=[]  ClampingZeroOutMax=[]  FilterDenConstantOutDataTypeStr=Inherit: Inherit via back propagation  FilterDenConstantOutMin=[]  FilterDenConstantOutMax=[]  PCopyOutDataTypeStr=Inherit: Inherit via back propagation  PCopyOutMin=[]  PCopyOutMax=[]  NCopyOutDataTypeStr=Inherit: Inherit via back propagation  NCopyOutMin=[]  NCopyOutMax=[]  IntegratorContinuousStateAttributes=''  IntegratorStateMustResolveToSignalObject=off  IntegratorRTWStateStorageClass=Auto  FilterContinuousStateAttributes=''  FilterStateMustResolveToSignalObject=off  FilterRTWStateStorageClass=Auto  ParallelPVariant=InternalParameters  IdealPVariant=Disabled  IVariant=InternalParameters  DVariant=InternalParameters  IntegratorVariant=Continuous  SatVariant=Disabled  AWVariant=Passthrough  PCopyVariant=Disabled  TRVariant=Disabled  FdbkBlocksVariant=Forward  IdealPFdbkVariant=Disabled  SatFdbkVariant=Disabled  DerivativeFilterVariant=ContFilter  NVariant=InternalParameters  NCopyVariant=Disabled  FilterICVariant=InternalICsFilter  IntegratorICVariant=InternalICs  ExternalResetVariant=Disabled  TRSumVariant=Passthrough  SumFdbkVariant=Disabled  SumVariant=Sum_PID  TsampFilterVariant=InternalTs  TsampNgainVariant=Passthrough  TsampIntegralVariant=Disabled_SignalSpec  ExternalSaturationOutDataTypeStr=Inherit: Same as second input  DerivativeSourceVariant=ErrorSignal  PreIntVariant=InternalPreInt
  Y PID Controller : slpidlib/PID Controller  Controller=PID  Form=Parallel  TimeDomain=Continuous-time  UseExternalTs=off  SampleTime=-1  IntegratorMethod=Forward Euler  FilterMethod=Forward Euler  ControllerParametersSource=internal  P=2  I=0  UseKiTs=off  D=1  UseExternalDerivativeSource=off  N=100  UseFilter=on  TunerSelectOption=Transfer Function Based (PID Tuner App)  InitialConditionSource=internal  InitialConditionForIntegrator=0  InitialConditionForFilter=0  DifferentiatorICPrevScaledInput=0  ExternalReset=none  TrackingMode=off  Kt=1  LimitOutput=off  SatLimitsSource=internal  UpperSaturationLimit=2  LowerSaturationLimit=-2  LinearizeAsGain=on  AntiWindupMode=none  Kb=1  LimitIntegrator=off  UpperIntegratorSaturationLimit=inf  LowerIntegratorSaturationLimit=-inf  POutMin=[]  POutMax=[]  IOutMin=[]  IOutMax=[]  DOutMin=[]  DOutMax=[]  NOutMin=[]  NOutMax=[]  SumOutMin=[]  SumOutMax=[]  SaturationOutMin=[]  SaturationOutMax=[]  PParamMin=[]  PParamMax=[]  IParamMin=[]  IParamMax=[]  DParamMin=[]  DParamMax=[]  NParamMin=[]  NParamMax=[]  KbParamMin=[]  KbParamMax=[]  KtParamMin=[]  KtParamMax=[]  KbOutMin=[]  KbOutMax=[]  KtOutMin=[]  KtOutMax=[]  IntegratorOutMin=[]  IntegratorOutMax=[]  FilterOutMin=[]  FilterOutMax=[]  SumI1OutMin=[]  SumI1OutMax=[]  SumI2OutMin=[]  SumI2OutMax=[]  SumI3OutMin=[]  SumI3OutMax=[]  SumI4OutMin=[]  SumI4OutMax=[]  SumDOutMin=[]  SumDOutMax=[]  DifferentiatorOutMin=[]  DifferentiatorOutMax=[]  FilterDiffOutCoefMin=[]  FilterDiffOutCoefMax=[]  ReciprocalOutMin=[]  ReciprocalOutMax=[]  SumDenOutMin=[]  SumDenOutMax=[]  SumNumOutMin=[]  SumNumOutMax=[]  DivideOutMin=[]  DivideOutMax=[]  UdiffTsProdOutMin=[]  UdiffTsProdOutMax=[]  NTsProdOutMin=[]  NTsProdOutMax=[]  UintegralTsProdOutMin=[]  UintegralTsProdOutMax=[]  UngainTsProdOutMin=[]  UngainTsProdOutMax=[]  ClampingZeroOutDataTypeStr=Inherit: Inherit via back propagation  ClampingZeroOutMin=[]  ClampingZeroOutMax=[]  FilterDenConstantOutDataTypeStr=Inherit: Inherit via back propagation  FilterDenConstantOutMin=[]  FilterDenConstantOutMax=[]  PCopyOutDataTypeStr=Inherit: Inherit via back propagation  PCopyOutMin=[]  PCopyOutMax=[]  NCopyOutDataTypeStr=Inherit: Inherit via back propagation  NCopyOutMin=[]  NCopyOutMax=[]  IntegratorContinuousStateAttributes=''  IntegratorStateMustResolveToSignalObject=off  IntegratorRTWStateStorageClass=Auto  FilterContinuousStateAttributes=''  FilterStateMustResolveToSignalObject=off  FilterRTWStateStorageClass=Auto  ParallelPVariant=InternalParameters  IdealPVariant=Disabled  IVariant=InternalParameters  DVariant=InternalParameters  IntegratorVariant=Continuous  SatVariant=Disabled  AWVariant=Passthrough  PCopyVariant=Disabled  TRVariant=Disabled  FdbkBlocksVariant=Forward  IdealPFdbkVariant=Disabled  SatFdbkVariant=Disabled  DerivativeFilterVariant=ContFilter  NVariant=InternalParameters  NCopyVariant=Disabled  FilterICVariant=InternalICsFilter  IntegratorICVariant=InternalICs  ExternalResetVariant=Disabled  TRSumVariant=Passthrough  SumFdbkVariant=Disabled  SumVariant=Sum_PID  TsampFilterVariant=InternalTs  TsampNgainVariant=Passthrough  TsampIntegralVariant=Disabled_SignalSpec  ExternalSaturationOutDataTypeStr=Inherit: Same as second input  DerivativeSourceVariant=ErrorSignal  PreIntVariant=InternalPreInt
  Z PID Controller : slpidlib/PID Controller  Controller=PID  Form=Parallel  TimeDomain=Continuous-time  UseExternalTs=off  SampleTime=-1  IntegratorMethod=Forward Euler  FilterMethod=Forward Euler  ControllerParametersSource=internal  P=1  I=1  UseKiTs=off  D=0.1  UseExternalDerivativeSource=off  N=100  UseFilter=on  TunerSelectOption=Transfer Function Based (PID Tuner App)  InitialConditionSource=internal  InitialConditionForIntegrator=0  InitialConditionForFilter=0  DifferentiatorICPrevScaledInput=0  ExternalReset=none  TrackingMode=off  Kt=1  LimitOutput=off  SatLimitsSource=internal  UpperSaturationLimit=3  LowerSaturationLimit=-3  LinearizeAsGain=on  AntiWindupMode=none  Kb=1  LimitIntegrator=off  UpperIntegratorSaturationLimit=inf  LowerIntegratorSaturationLimit=-inf  POutMin=[]  POutMax=[]  IOutMin=[]  IOutMax=[]  DOutMin=[]  DOutMax=[]  NOutMin=[]  NOutMax=[]  SumOutMin=[]  SumOutMax=[]  SaturationOutMin=[]  SaturationOutMax=[]  PParamMin=[]  PParamMax=[]  IParamMin=[]  IParamMax=[]  DParamMin=[]  DParamMax=[]  NParamMin=[]  NParamMax=[]  KbParamMin=[]  KbParamMax=[]  KtParamMin=[]  KtParamMax=[]  KbOutMin=[]  KbOutMax=[]  KtOutMin=[]  KtOutMax=[]  IntegratorOutMin=[]  IntegratorOutMax=[]  FilterOutMin=[]  FilterOutMax=[]  SumI1OutMin=[]  SumI1OutMax=[]  SumI2OutMin=[]  SumI2OutMax=[]  SumI3OutMin=[]  SumI3OutMax=[]  SumI4OutMin=[]  SumI4OutMax=[]  SumDOutMin=[]  SumDOutMax=[]  DifferentiatorOutMin=[]  DifferentiatorOutMax=[]  FilterDiffOutCoefMin=[]  FilterDiffOutCoefMax=[]  ReciprocalOutMin=[]  ReciprocalOutMax=[]  SumDenOutMin=[]  SumDenOutMax=[]  SumNumOutMin=[]  SumNumOutMax=[]  DivideOutMin=[]  DivideOutMax=[]  UdiffTsProdOutMin=[]  UdiffTsProdOutMax=[]  NTsProdOutMin=[]  NTsProdOutMax=[]  UintegralTsProdOutMin=[]  UintegralTsProdOutMax=[]  UngainTsProdOutMin=[]  UngainTsProdOutMax=[]  ClampingZeroOutDataTypeStr=Inherit: Inherit via back propagation  ClampingZeroOutMin=[]  ClampingZeroOutMax=[]  FilterDenConstantOutDataTypeStr=Inherit: Inherit via back propagation  FilterDenConstantOutMin=[]  FilterDenConstantOutMax=[]  PCopyOutDataTypeStr=Inherit: Inherit via back propagation  PCopyOutMin=[]  PCopyOutMax=[]  NCopyOutDataTypeStr=Inherit: Inherit via back propagation  NCopyOutMin=[]  NCopyOutMax=[]  IntegratorContinuousStateAttributes=''  IntegratorStateMustResolveToSignalObject=off  IntegratorRTWStateStorageClass=Auto  FilterContinuousStateAttributes=''  FilterStateMustResolveToSignalObject=off  FilterRTWStateStorageClass=Auto  ParallelPVariant=InternalParameters  IdealPVariant=Disabled  IVariant=InternalParameters  DVariant=InternalParameters  IntegratorVariant=Continuous  SatVariant=Disabled  AWVariant=Passthrough  PCopyVariant=Disabled  TRVariant=Disabled  FdbkBlocksVariant=Forward  IdealPFdbkVariant=Disabled  SatFdbkVariant=Disabled  DerivativeFilterVariant=ContFilter  NVariant=InternalParameters  NCopyVariant=Disabled  FilterICVariant=InternalICsFilter  IntegratorICVariant=InternalICs  ExternalResetVariant=Disabled  TRSumVariant=Passthrough  SumFdbkVariant=Disabled  SumVariant=Sum_PID  TsampFilterVariant=InternalTs  TsampNgainVariant=Passthrough  TsampIntegralVariant=Disabled_SignalSpec  ExternalSaturationOutDataTypeStr=Inherit: Same as second input  DerivativeSourceVariant=ErrorSignal  PreIntVariant=InternalPreInt
  Global Desired Vel. : Outport
  wires:
  Demux1/1 -> X PID Controller/1
  Demux1/3 -> Z PID Controller/1
  Demux1/2 -> Y PID Controller/1
  Pos._error/1 -> Demux1/1
  Mux/1 -> Scope/1, Global Desired Vel./1
  X PID Controller/1 -> Mux/1
  Y PID Controller/1 -> Mux/2
  Z PID Controller/1 -> Mux/3

== system V1/Q-filter ==
  In1 : Inport
  Demux8 : Demux  Outputs=3
  LTI System6 : cstblocks/LTI System  sys=tf([1],[1/1 1.414/1 1])  IC=[]  PadeOrder=0
  LTI System7 : cstblocks/LTI System  sys=tf([1],[1/1 1.414/1 1])  IC=[]  PadeOrder=0
  LTI System8 : cstblocks/LTI System  sys=tf([1],[1/1 1.414/1 1])  IC=[]  PadeOrder=0
  Mux13 : Mux  Inputs=3
  Out1 : Outport
  wires:
  LTI System8/1 -> Mux13/1
  Demux8/2 -> LTI System6/1
  Mux13/1 -> Out1/1
  Demux8/1 -> LTI System8/1
  In1/1 -> Demux8/1
  Demux8/3 -> LTI System7/1
  LTI System6/1 -> Mux13/2
  LTI System7/1 -> Mux13/3

== system V1/Translational Motion Dynamics ==
  Body Translational Force : Inport
  Euler_attitude : Inport  Port=2
  Coordinate Transformation Conversion : robotcorelib/Coordinate Transformation Conversion  InputRepresentation=Euler Angles  InputEulerSequence=XYZ  ShowTrVecInputPort=on  OutputRepresentation=Rotation Matrix  OutputEulerSequence=ZYX  ShowTrVecOutputPort=on  SimulateUsing=Interpreted execution
  Divide : Product  Inputs=*/
  Product1 : Product  Multiplication=Matrix(*)
  Scope : Scope
      settings: ActiveDisplayYMinimum=-1.03672  ActiveDisplayYMaximum=0.5142  DataLoggingVariableName=ScopeData8
  Scope1 : Scope
      settings: ActiveDisplayYMinimum=-79.44315  ActiveDisplayYMaximum=8.82783  DataLoggingVariableName=ScopeData9
  Sum1 : Sum  Inputs=|++
  gravity : Constant  Value=[0;0;9.80665]
  Global Translational Accel. : Outport
  wires:
  Coordinate Transformation Conversion/1 -> Product1/1
  Sum1/1 -> Scope/1, Global Translational Accel./1  "Global Translational Accel."
  Euler_attitude/1 -> Coordinate Transformation Conversion/1
  Product1/1 -> Divide/1
  Divide/1 -> Sum1/1
  gravity/1 -> Sum1/2
  Body Translational Force/1 -> Scope1/1, Product1/2
  [Main_Vehicle_Mass] -> Divide/2
